simulink model "ExRobotAndEnvironmentControllerContPI.org"  (R2017a)
settings: Solver=ode45  StartTime=0.0  StopTime=1000  FixedStep=.01  RelTol=1e-3  EnableMultiTasking=on
values from neighbouring files (symbols this model uses):
  INITIAL_ROBOT_POS_THETA = 1.5*2    (= 3)    [InitRobotAndEnvironment.m]
  INITIAL_ROBOT_POS_X = 0    [InitRobotAndEnvironment.m]
  INITIAL_ROBOT_POS_Y = 0    [InitRobotAndEnvironment.m]
  INTER_WHEEL_DISTANCE = 0.12    [InitRobotAndEnvironment.m]
  ki_teta = omega*omega/alpha    (= 0.12)    [InitRobotAndEnvironment.m]
  kp_teta = 3*ksi*omega/alpha    (= 0.36)    [InitRobotAndEnvironment.m]
  MAX_SPEED = .5    (= 0.5)    [InitRobotAndEnvironment.m]
  Te = 0.05/w    [InitRobotAndEnvironment.m]
  ts = SENSOR_SAMPLING_TIME    (= 0.001)    [InitRobotAndEnvironment.m]
  ts_anim = ANIMATION_SAMPLING_TIME    (= 0.01)    [InitRobotAndEnvironment.m]
undefined symbols (not defined in the file or in its folder): Env, Robot, RobotInit
settings Model: Creator=alex  LastModifiedBy=cathrind
settings DataIOCC: LimitDataPoints=on  SaveFormat=Array  SignalLoggingSaveFormat=ModelDataLogs
settings OptimizationCC: ExpressionDepthLimit=2147483647  LifeSpan=inf
settings DebuggingCC: UnderspecifiedInitializationDetection=Classic  MergeDetectMultiDrivingBlocksExec=none  FcnCallInpInsideContextMsg=warning  StateNameClashWarn=warning  SFUnexpectedBacktrackingDiag=warning  SFNoUnconditionalDefaultTransitionDiag=warning  SFExecutionAtInitializationDiag=none
settings HardwareCC: ProdBitPerPointer=32  ProdBitPerSizeT=32  ProdBitPerPtrDiffT=32  ProdLargestAtomicFloat=None  ProdIntDivRoundTo=Undefined  ProdEndianess=Unspecified  ProdWordSize=32  ProdHWDeviceType=32-bit Generic
settings ModelReferenceCC: PropagateSignalLabelsOutOfModel=off
settings SFSimCC: SimParseCustomCode=off
settings GRTTargetCC: TargetLangStandard=C89/C90 (ANSI)  GeneratePreprocessorConditionals=Disable all  CombineOutputUpdateFcns=off  GRTInterface=on
settings ConfigComp: CovMetricSettings=dw  CovHtmlReporting=on  CovSaveCumulativeToWorkspaceVar=on  CovSaveSingleToWorkspaceVar=on  CovExternalEMLEnable=off

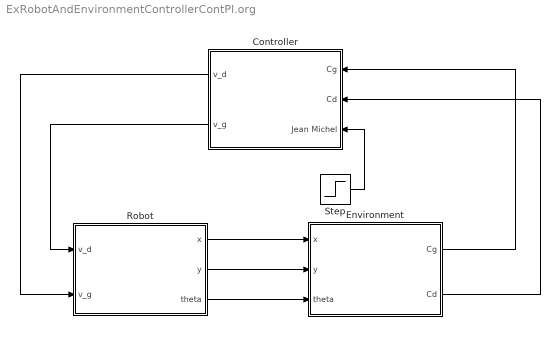
== system ExRobotAndEnvironmentControllerContPI.org ==
  Controller : Subsystem
  Environment : Subsystem
  Robot : Subsystem
  Step : Step  Time=3  Before=1000  After=0  SampleTime=Te
  wires:
  Robot/1(x) -> Environment/1(x)
  Robot/2(y) -> Environment/2(y)
  Robot/3(theta) -> Environment/3(theta)
  Environment/1(Cg) -> Controller/1(Cg)
  Environment/2(Cd) -> Controller/2(Cd)
  Controller/1(v_d) -> Robot/2(v_g)
  Controller/2(v_g) -> Robot/1(v_d)
  Step/1 -> Controller/3(Jean Michel)

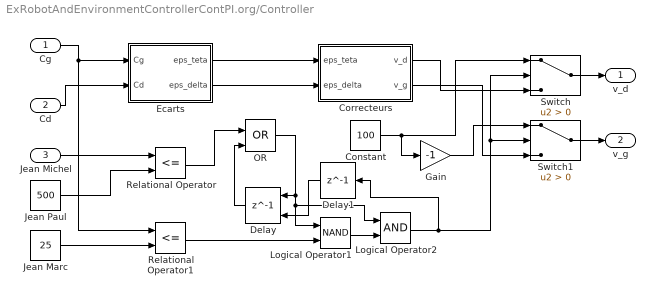
== system ExRobotAndEnvironmentControllerContPI.org/Controller ==
  Cg : Inport
  Cd : Inport  Port=2
  Jean Michel : Inport  Port=3
  Constant : Constant  Value=100
  "Correcteurs " : Subsystem
  Delay : Delay  DelayLength=1  InitialCondition=0  ExternalReset=Falling  SampleTime=Te
      settings: InputPortMap=u0,r5
  Delay1 : Delay  DelayLength=1  InitialCondition=0  SampleTime=Te
  Ecarts : Subsystem
  Gain : Gain  Gain=-1
  Jean Marc : Constant  Value=25
  Jean Paul : Constant  Value=500
  Logical Operator1 : Logic  Operator=NAND  AllPortsSameDT=off  OutDataTypeStr=boolean
  Logical Operator2 : Logic  AllPortsSameDT=off  OutDataTypeStr=boolean
  OR : Logic  Operator=OR  IconShape=distinctive  AllPortsSameDT=off  OutDataTypeStr=boolean
  Relational Operator : RelationalOperator  Operator=<=  OutDataTypeStr=boolean  RndMeth=Simplest
  Relational Operator1 : RelationalOperator  Operator=<=  OutDataTypeStr=boolean  RndMeth=Simplest
  Switch : Switch  Criteria=u2 > Threshold
  Switch1 : Switch  Criteria=u2 > Threshold
  v_d : Outport
  v_g : Outport  Port=2
  wires:
  Ecarts/2(eps_delta) -> "Correcteurs "/2(eps_delta)
  Cg/1 -> Relational Operator1/1, Ecarts/1(Cg)
  Cd/1 -> Ecarts/2(Cd)
  Ecarts/1(eps_teta) -> "Correcteurs "/1(eps_teta)
  Switch/1 -> v_d/1
  Switch1/1 -> v_g/1
  Constant/1 -> Switch/1, Gain/1
  Jean Michel/1 -> Relational Operator/1
  Jean Paul/1 -> Relational Operator/2
  Jean Marc/1 -> Relational Operator1/2
  Relational Operator/1 -> OR/1
  Delay/1 -> OR/2
  OR/1 -> Logical Operator2/1, Logical Operator1/1, Delay/1
  Logical Operator1/1 -> Logical Operator2/2
  Relational Operator1/1 -> Logical Operator1/2
  Logical Operator2/1 -> Delay1/1, Switch/2, Switch1/2
  "Correcteurs "/1(v_d) -> Switch/3
  Gain/1 -> Switch1/1
  "Correcteurs "/2(v_g) -> Switch1/3
  Delay1/1 -> Delay/2

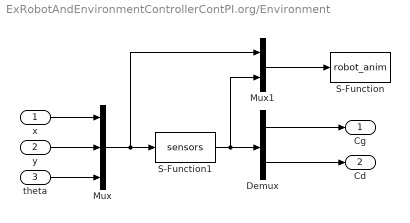
== system ExRobotAndEnvironmentControllerContPI.org/Environment ==
  x : Inport
  y : Inport  Port=2
  theta : Inport  Port=3
  Demux : Demux  Outputs=2
  Mux : Mux  Inputs=3
  Mux1 : Mux  Inputs=2
  S-Function : S-Function  FunctionName=robot_anim  Parameters=ts_anim,Env,Robot,RobotInit  SFunctionDeploymentMode=off  EnableBusSupport=off
  S-Function1 : S-Function  FunctionName=sensors  Parameters=ts,Env,Robot  SFunctionDeploymentMode=off  EnableBusSupport=off
  Cg : Outport
  Cd : Outport  Port=2
  wires:
  x/1 -> Mux/1
  y/1 -> Mux/2
  theta/1 -> Mux/3
  Mux/1 -> S-Function1/1, Mux1/1
  S-Function1/1 -> Mux1/2, Demux/1
  Mux1/1 -> S-Function/1
  Demux/1 -> Cg/1
  Demux/2 -> Cd/1

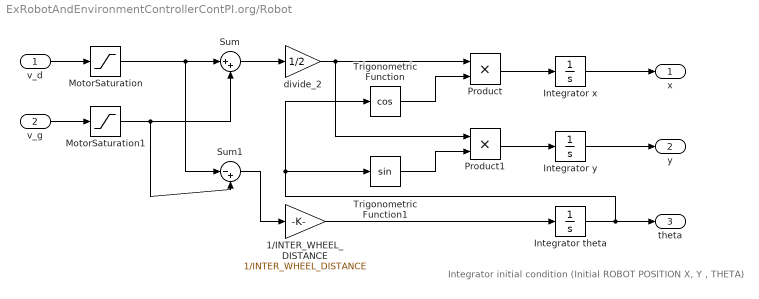
== system ExRobotAndEnvironmentControllerContPI.org/Robot ==
  note: Integrator initial condition (Initial ROBOT POSITION X, Y , THETA)
  v_d : Inport
  v_g : Inport  Port=2
  1/INTER_WHEEL_DISTANCE : Gain  Gain=1/INTER_WHEEL_DISTANCE
  Integrator theta : Integrator  InitialCondition=INITIAL_ROBOT_POS_THETA
  Integrator x : Integrator  InitialCondition=INITIAL_ROBOT_POS_X
  Integrator y : Integrator  InitialCondition=INITIAL_ROBOT_POS_Y
  MotorSaturation : Saturate  UpperLimit=MAX_SPEED  LowerLimit=-MAX_SPEED
  MotorSaturation1 : Saturate  UpperLimit=MAX_SPEED  LowerLimit=-MAX_SPEED
  Product : Product  RndMeth=Zero
  Product1 : Product  RndMeth=Zero
  Sum : Sum  Inputs=|++
  Sum1 : Sum  Inputs=|-+
  Trigonometric Function : Trigonometry  Operator=cos
  Trigonometric Function1 : Trigonometry
  divide_2 : Gain  Gain=1/2
  x : Outport
  y : Outport  Port=2
  theta : Outport  Port=3
  wires:
  v_d/1 -> MotorSaturation/1
  Integrator x/1 -> x/1
  Integrator y/1 -> y/1
  Integrator theta/1 -> Trigonometric Function/1, Trigonometric Function1/1, theta/1
  Sum/1 -> divide_2/1
  divide_2/1 -> Product1/1, Product/1
  Trigonometric Function/1 -> Product/2
  Trigonometric Function1/1 -> Product1/2
  Product/1 -> Integrator x/1
  Product1/1 -> Integrator y/1
  Sum1/1 -> 1/INTER_WHEEL_DISTANCE/1
  1/INTER_WHEEL_DISTANCE/1 -> Integrator theta/1
  v_g/1 -> MotorSaturation1/1
  MotorSaturation1/1 -> Sum/2, Sum1/2
  MotorSaturation/1 -> Sum/1, Sum1/1

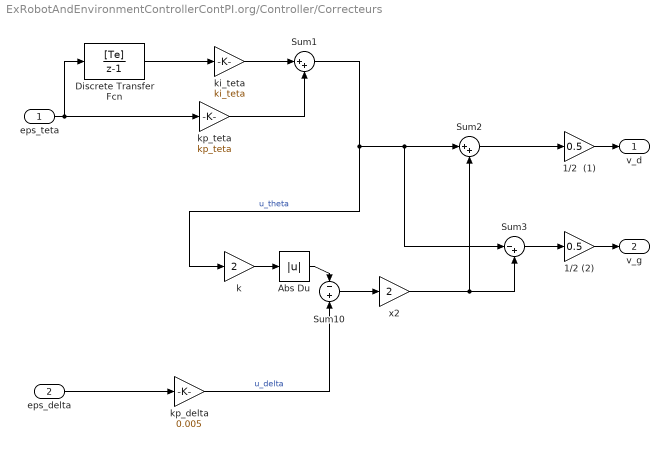
== system ExRobotAndEnvironmentControllerContPI.org/Controller/Correcteurs  ==
  eps_teta : Inport
  eps_delta : Inport  Port=2
  1/2  (1) : Gain  Gain=0.5  SaturateOnIntegerOverflow=on  OutDataTypeStr=Inherit: Same as input  ParamDataTypeStr=Inherit: Same as input
  1/2 (2) : Gain  Gain=0.5  SaturateOnIntegerOverflow=on  OutDataTypeStr=Inherit: Same as input  ParamDataTypeStr=Inherit: Same as input
  Abs Du : Abs  SaturateOnIntegerOverflow=on
  Discrete Transfer Fcn : DiscreteTransferFcn  Numerator=[Te]  Denominator=[1 -1]  SampleTime=Te
  Sum1 : Sum  Inputs=|++  SaturateOnIntegerOverflow=on
  Sum10 : Sum  Inputs=-+  SaturateOnIntegerOverflow=on
  Sum2 : Sum  Inputs=|++  SaturateOnIntegerOverflow=on
  Sum3 : Sum  Inputs=|-+  SaturateOnIntegerOverflow=on
  k : Gain  Gain=2  SaturateOnIntegerOverflow=on  OutDataTypeStr=Inherit: Same as input  ParamDataTypeStr=Inherit: Same as input
  ki_teta : Gain  Gain=ki_teta  SaturateOnIntegerOverflow=on  OutDataTypeStr=Inherit: Same as input  ParamDataTypeStr=Inherit: Same as input
  kp_delta : Gain  Gain=0.005
  kp_teta : Gain  Gain=kp_teta  SaturateOnIntegerOverflow=on  OutDataTypeStr=Inherit: Same as input  ParamDataTypeStr=Inherit: Same as input
  x2 : Gain  Gain=2  SaturateOnIntegerOverflow=on  OutDataTypeStr=Inherit: Same as input  ParamDataTypeStr=Inherit: Same as input
  v_d : Outport
  v_g : Outport  Port=2
  wires:
  ki_teta/1 -> Sum1/1
  kp_teta/1 -> Sum1/2
  Sum2/1 -> 1/2  (1)/1
  Sum3/1 -> 1/2 (2)/1
  k/1 -> Abs Du/1
  kp_delta/1 -> Sum10/2  "u_delta"
  eps_teta/1 -> Discrete Transfer Fcn/1, kp_teta/1
  Abs Du/1 -> Sum10/1
  x2/1 -> Sum2/2, Sum3/2
  Sum10/1 -> x2/1
  Sum1/1 -> k/1, Sum2/1, Sum3/1  "u_theta"
  1/2  (1)/1 -> v_d/1
  1/2 (2)/1 -> v_g/1
  eps_delta/1 -> kp_delta/1
  Discrete Transfer Fcn/1 -> ki_teta/1

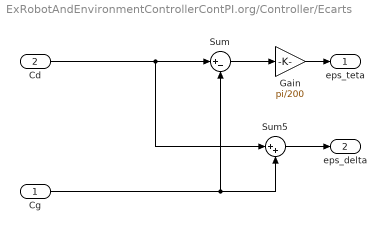
== system ExRobotAndEnvironmentControllerContPI.org/Controller/Ecarts ==
  Cg : Inport
  Cd : Inport  Port=2
  Gain : Gain  Gain=pi/200
  Sum : Sum  Inputs=|+-
  Sum5 : Sum  Inputs=|++
  eps_teta : Outport
  eps_delta : Outport  Port=2
  wires:
  Sum/1 -> Gain/1
  Cd/1 -> Sum/1, Sum5/1
  Cg/1 -> Sum/2, Sum5/2
  Gain/1 -> eps_teta/1
  Sum5/1 -> eps_delta/1
